simulink model "MultirotorModel"  (R2024b)
settings: Solver=VariableStepAuto  StartTime=0.0  StopTime=simTime  FixedStep=0.001  RelTol=1e-3  EnableMultiTasking=on
undefined symbols (not defined in the file): baseMission, bird_cycle, bird_end, bird_start, Controller, ctrl_mass, ctrl_thrust_perturbation_param, DiscIntNeverNeededParam, Dz, Earth, Gravity, initialConditions, Iz, mass_param, Nz, Pz, startFlightTime, UAVSampleTime, Vehicle, WGS84
libraries: slpidlib x10, uavalgslib x6, simulink x3, sharedutil x2, aerolibconvert2 x2, aerolibtransform2 x2, robotcorelib x1, uavutilslib x1, shared6dof x1, aerolibasang x1, sensorinslib x1
(part 3 of 3)

== system MultirotorModel/Inner Loop and Plant Model/High-FidelityModel/Control System/Controller/gravity feedforward//equilibrium thrust ==
  note: Derived from the work by Sertac Karaman and Fabian Riether
  note: ALTITUDE
  states_estim : Inport
  PosZ : Inport  Port=2
  Bus Selector1 : BusSelector  OutputSignals=pos_vel.z,pos_vel.vz
  D_z1 : Gain  Gain=3.5  ParamDataTypeStr=single  OutDataTypeStr=single  SaturateOnIntegerOverflow=on
  Discrete-Time Integrator : DiscreteIntegrator  SampleTime=UAVSampleTime  LimitOutput=on  UpperSaturationLimit=2  LowerSaturationLimit=-2  ICPrevOutput=DiscIntNeverNeededParam  ICPrevScaledInput=DiscIntNeverNeededParam
  I_pr : Gain  Gain=0.1
  MPC_THR_HOVER : Constant  Value=-Gravity*ctrl_mass  OutDataTypeStr=single
  P_z1 : Gain  Gain=0.4  ParamDataTypeStr=single  OutDataTypeStr=single  SaturateOnIntegerOverflow=on
  SaturationThrust1 : Saturate  UpperLimit=63  LowerLimit=-63  OutDataTypeStr=single
  SaturationThrust2 : Saturate  Commented=on  UpperLimit=4*Controller.totalThrustMaxRelative*Controller.motorsThrustPerMotorMax  LowerLimit=-4*Controller.totalThrustMaxRelative*Controller.motorsThrustPerMotorMax  OutDataTypeStr=single
  Scope : Scope
  Sum1 : Sum  Inputs=++-  OutDataTypeStr=single  AccumDataTypeStr=single  SaturateOnIntegerOverflow=on
  Sum2 : Sum  Inputs=+-|  OutDataTypeStr=single  AccumDataTypeStr=single  SaturateOnIntegerOverflow=on
  Sum5 : Sum  Inputs=++|  OutDataTypeStr=single  AccumDataTypeStr=single  SaturateOnIntegerOverflow=on
  altitude_cmd : Outport  VectorParamsAs1DForOutWhenUnconnected=off
  wires:
  I_pr/1 -> Discrete-Time Integrator/1
  Discrete-Time Integrator/1 -> Sum1/1
  D_z1/1 -> Sum1/3  "dz"
  Sum2/1 -> I_pr/1, P_z1/1  "pitch/roll error"
  Bus Selector1/2 -> D_z1/1  "<vz>"
  P_z1/1 -> Sum1/2
  states_estim/1 -> Bus Selector1/1
  Bus Selector1/1 -> Sum2/2  "<z>"
  PosZ/1 -> Sum2/1
  Sum1/1 -> Sum5/2
  Sum5/1 -> Scope/1, SaturationThrust1/1
  MPC_THR_HOVER/1 -> Sum5/1
  SaturationThrust1/1 -> altitude_cmd/1

== system MultirotorModel/Inner Loop and Plant Model/High-FidelityModel/Control System/Controller/thrustsToMotorCommands ==
  thrusts_refin : Inport
  MotorDirections : Gain  Gain=[1 -1 1 -1]
  Saturation5 : Saturate  Commented=on  UpperLimit=Vehicle.Motor.maxLimit  LowerLimit=Vehicle.Motor.minLimit
  ThrustToMotorCommand : Gain  Gain=-Vehicle.Motor.thrustToMotorCommand
  motors_cmdout : Outport  VectorParamsAs1DForOutWhenUnconnected=off
  wires:
  MotorDirections/1 -> motors_cmdout/1
  thrusts_refin/1 -> ThrustToMotorCommand/1
  ThrustToMotorCommand/1 -> MotorDirections/1

== system MultirotorModel/Inner Loop and Plant Model/High-FidelityModel/Plant Model/AC model/Applied Force Calculation ==
  gravity force : Inport  Unit=N
  Aerodynamic Forces : Inport  Port=2  Unit=N
  Motor Forces : Inport  Port=3  Unit=N
  Add1 : Sum  Inputs=+++
  Signal Specification : SignalSpecification  Dimensions=3
  External Forces : Outport  Unit=N  VectorParamsAs1DForOutWhenUnconnected=off
  wires:
  Add1/1 -> Signal Specification/1
  Motor Forces/1 -> Add1/3  "Motor Thrust"
  Aerodynamic Forces/1 -> Add1/2
  gravity force/1 -> Add1/1
  Signal Specification/1 -> External Forces/1

== system MultirotorModel/Inner Loop and Plant Model/High-FidelityModel/Plant Model/AC model/Drag Calculation ==
  Density : Inport  Unit=kg/m^3
  Vb : Inport  Port=2  Unit=m/second
  Drag Calc : Subsystem
  Gain3 : Gain  Gain=-1
  Product : Product  RndMeth=Zero
  Sign : Signum  ZeroCross=off
  Drag : Outport  Unit=N  VectorParamsAs1DForOutWhenUnconnected=off
  wires:
  Density/1 -> Drag Calc/1(Density)
  Sign/1 -> Gain3/1
  Drag Calc/1(drag) -> Product/1
  Gain3/1 -> Product/2
  Product/1 -> Drag/1  "xDrag"
  Vb/1 -> Sign/1, Drag Calc/2(vel)

== system MultirotorModel/Inner Loop and Plant Model/High-FidelityModel/Plant Model/AC model/Gravity Force Calculation ==
  DCMbe : Inport
  gravity : Inport  Port=2  Unit=m/s^2
  Gain1 : Gain  Gain=ctrl_mass
  Product : Product  Multiplication=Matrix(*)
  gravity force : Outport  Unit=N  VectorParamsAs1DForOutWhenUnconnected=off
  wires:
  gravity/1 -> Gain1/1
  Gain1/1 -> Product/2  "gravity force NED"
  Product/1 -> gravity force/1
  DCMbe/1 -> Product/1

== system MultirotorModel/Inner Loop and Plant Model/High-FidelityModel/Plant Model/AC model/Motor Forces and Torques ==
  Vb : Inport
  Density : Inport  Port=2
  pqr : Inport  Port=3
  Motor Commands : Inport  Port=4
  D1 : Constant  Value=[Vehicle.Airframe.xy -Vehicle.Airframe.xy Vehicle.Airframe.h]
  D2 : Constant  Value=[Vehicle.Airframe.xy Vehicle.Airframe.xy Vehicle.Airframe.h]
  D3 : Constant  Value=[-Vehicle.Airframe.xy Vehicle.Airframe.xy Vehicle.Airframe.h]
  D4 : Constant  Value=[-Vehicle.Airframe.xy -Vehicle.Airframe.xy Vehicle.Airframe.h]
  For Each Subsystem : Subsystem  TreatAsAtomicUnit=on
  MotorsToW : Subsystem
  Sum of Elements : Sum  Inputs=+  CollapseMode=Specified dimension  CollapseDim=2
  Sum of Elements1 : Sum  Inputs=+  CollapseMode=Specified dimension  CollapseDim=2
  Vector Concatenate : Concatenate  NumInputs=4  Mode=Multidimensional array  ConcatenateDimension=2
  Motor Forces : Outport  Unit=N  VectorParamsAs1DForOutWhenUnconnected=off
  Motor Torques : Outport  Port=2  Unit=N*m  VectorParamsAs1DForOutWhenUnconnected=off
  wires:
  D4/1 -> Vector Concatenate/4
  MotorsToW/1(omegas_datout) -> For Each Subsystem/4(w)
  Vector Concatenate/1 -> For Each Subsystem/5(D)
  For Each Subsystem/2(Moments) -> Sum of Elements1/1
  pqr/1 -> For Each Subsystem/3(Omega)
  Vb/1 -> For Each Subsystem/1(Vb)
  Motor Commands/1 -> MotorsToW/1(motors_datin)
  D1/1 -> Vector Concatenate/1
  D3/1 -> Vector Concatenate/3
  D2/1 -> Vector Concatenate/2
  Sum of Elements1/1 -> Motor Torques/1
  Density/1 -> For Each Subsystem/2(rho)
  Sum of Elements/1 -> Motor Forces/1
  For Each Subsystem/1(Forces) -> Sum of Elements/1

== system MultirotorModel/Inner Loop and Plant Model/High-FidelityModel/Plant Model/Bus setup/Generate GPS Data ==
  XYZ (NEU) : Inport
  "Vx, Vy, Vz" : Inport  Port=2
  DCM : Inport  Port=3
  GPS Model : sensorinslib/INS  MountingLocation=[0 0 0]  RollAccuracy=0.2  PitchAccuracy=0.2  YawAccuracy=1  PositionAccuracy=0.85  VelocityAccuracy=0.05  UseAccelAndAngVel=off  AccelerationAccuracy=0  AngularVelocityAccuracy=0  TimeInput=off  PositionErrorFactor=[0 0 0]  SeedDouble=67  SimulateUsing=Code generation
  Reshape : Reshape  OutputDimensionality=Customize  OutputDimensions=[1 3]
  Reshape1 : Reshape  OutputDimensionality=Customize  OutputDimensions=[1 3]
  "Scale and Assemble GPS Data " : Subsystem
  Terminator1 : Terminator
  Variant Source : VariantSource  VariantControlMode=label  LabelModeActiveChoice=Model
  Variant Source1 : VariantSource  VariantControlMode=label  LabelModeActiveChoice=Model
  GPSData : Outport  VectorParamsAs1DForOutWhenUnconnected=off
  wires:
  DCM/1 -> GPS Model/3
  "Vx, Vy, Vz"/1 -> Variant Source1/1, Reshape1/1
  XYZ (NEU)/1 -> Variant Source/1, Reshape/1
  GPS Model/3 -> Terminator1/1
  Reshape/1 -> GPS Model/1
  Reshape1/1 -> GPS Model/2
  "Scale and Assemble GPS Data "/1(Out1) -> GPSData/1
  GPS Model/1 -> Variant Source/2
  Variant Source1/1 -> "Scale and Assemble GPS Data "/2(Ve)
  GPS Model/2 -> Variant Source1/2
  Variant Source/1 -> "Scale and Assemble GPS Data "/1(Xe)

== system MultirotorModel/Guidance Logic/Full Guidance Logic/Guidance Stateflow/Guidance Mode Selector/GuidanceLogic.WP/Dist2WP/Subsystem ==
  V : Inport
  Dot Product1 : DotProduct  OutDataTypeStr=Inherit: Inherit via internal rule
  Product : Product  Inputs=*/
  Saturation : Saturate  UpperLimit=inf  LowerLimit=0.00001
  Sqrt : Sqrt
  V_unit : Outport
  wires:
  V/1 -> Dot Product1/2, Dot Product1/1, Product/1
  Sqrt/1 -> Product/2
  Dot Product1/1 -> Saturation/1
  Saturation/1 -> Sqrt/1
  Product/1 -> V_unit/1

== system MultirotorModel/Inner Loop and Plant Model/High-FidelityModel/Plant Model/AC model/Drag Calculation/Drag Calc ==
  Density : Inport  Unit=kg/m^3
  vel : Inport  Port=2  Unit=m/s
  Dynamic Pressure : aerolibasang/Dynamic Pressure
  Gain : Gain  Gain=[.25 .25]
  Mux1 : Mux  Inputs=2
  Product : Product  Inputs=3  RndMeth=Zero
  diameter : Constant  Value=0.65  SampleTime=0
  dragCoeff : Constant  Value=Vehicle.Airframe.Cdx  SampleTime=0
  drag : Outport  Unit=N  VectorParamsAs1DForOutWhenUnconnected=off
  wires:
  Product/1 -> drag/1
  dragCoeff/1 -> Product/3  "Cd"
  Dynamic Pressure/1 -> Product/1  "q"
  diameter/1 -> Gain/1, Mux1/2
  Mux1/1 -> Product/2  "S"
  Gain/1 -> Mux1/1
  vel/1 -> Dynamic Pressure/1
  Density/1 -> Dynamic Pressure/2

== system MultirotorModel/Inner Loop and Plant Model/High-FidelityModel/Plant Model/AC model/Motor Forces and Torques/For Each Subsystem ==
  Vb : Inport  PortDimensions=3
  rho : Inport  Port=2  PortDimensions=1
  Omega : Inport  Port=3
  w : Inport  Port=4  Partition=on  PartitionDimension=2  PartitionWidth=1  PartitionOffset=0
  D : Inport  Port=5  Partition=on  PartitionDimension=2  PartitionWidth=1  PartitionOffset=0
  For Each : ForEach  DisableCoverage=on
  RotorDynamics : Subsystem  TreatAsAtomicUnit=on
      mask init:
      | aeroicon('aeroblk');
      settings: RTWFcnNameOpts=Use subsystem name  RTWFileNameOpts=Use function name
  Forces : Outport  ConcatenationDimension=2  VectorParamsAs1DForOutWhenUnconnected=off
  Moments : Outport  Port=2  ConcatenationDimension=2  VectorParamsAs1DForOutWhenUnconnected=off
  wires:
  RotorDynamics/1(Fxyz) -> Forces/1
  RotorDynamics/2(Mxyz) -> Moments/1
  Vb/1 -> RotorDynamics/1(Vb)
  Omega/1 -> RotorDynamics/2(pqr)
  rho/1 -> RotorDynamics/3(rho)
  D/1 -> RotorDynamics/5(Arm)
  w/1 -> RotorDynamics/4(w)

== system MultirotorModel/Inner Loop and Plant Model/High-FidelityModel/Plant Model/AC model/Motor Forces and Torques/MotorsToW ==
  motors_datin : Inport
  Motordirections : Gain  Gain=[1 -1 1 -1]  ParamDataTypeStr=single  OutDataTypeStr=Inherit: Inherit via back propagation  SaturateOnIntegerOverflow=on
  Motordirections1 : Gain  Gain=[1 -1 1 -1]  ParamDataTypeStr=single  OutDataTypeStr=Inherit: Inherit via back propagation  SaturateOnIntegerOverflow=on
  Saturation1 : Saturate  UpperLimit=99999999999  LowerLimit=1  OutDataTypeStr=Inherit: Inherit via back propagation
  Saturation5 : Saturate  Commented=on  UpperLimit=Vehicle.Motor.maxLimit  LowerLimit=Vehicle.Motor.minLimit  OutDataTypeStr=Inherit: Inherit via back propagation
  Signed Sqrt : Sqrt  Operator=signedSqrt  OutDataTypeStr=Inherit: Inherit via back propagation
  motorsToW2_Gain : Gain  Gain=Vehicle.Motor.commandToW2Gain  ParamDataTypeStr=single  OutDataTypeStr=Inherit: Inherit via back propagation  SaturateOnIntegerOverflow=on
  omegas_datout : Outport  VectorParamsAs1DForOutWhenUnconnected=off
  wires:
  motorsToW2_Gain/1 -> Signed Sqrt/1
  Motordirections1/1 -> motorsToW2_Gain/1
  Signed Sqrt/1 -> omegas_datout/1
  motors_datin/1 -> Motordirections/1
  Motordirections/1 -> Saturation1/1
  Saturation1/1 -> Motordirections1/1

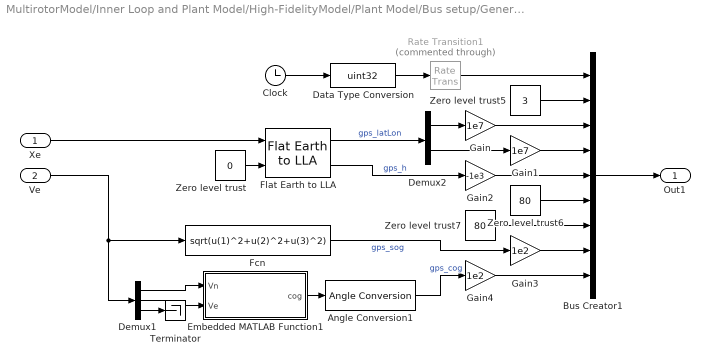
== system MultirotorModel/Inner Loop and Plant Model/High-FidelityModel/Plant Model/Bus setup/Generate GPS Data/Scale and Assemble GPS Data  ==
  Xe : Inport
  Ve : Inport  Port=2
  Angle Conversion1 : aerolibconvert2/Angle Conversion  IU=rad  OU=deg
  Bus Creator1 : BusCreator  Inputs=9  OutDataTypeStr=Bus: gps_raw_int  NonVirtualBus=on
      settings: InheritFromInputs=off
  Clock : Clock
      settings: AttributesFormatString=Decimation: %<Decimation>
  Data Type Conversion : DataTypeConversion  OutDataTypeStr=uint32  SaturateOnIntegerOverflow=off  RndMeth=Floor
  Demux1 : Demux  Outputs=3
  Demux2 : Demux  Outputs=2
  Embedded MATLAB Function1 : MATLAB Function  TreatAsAtomicUnit=on
  Fcn : Fcn  Expr=sqrt(u(1)^2+u(2)^2+u(3)^2)
  Flat Earth to LLA : aerolibtransform2/Flat Earth to LLA  units=Metric (MKS)  ptype=Earth (WGS84)  F=1/298.257223563  R=6378137  refPosPort=off  LL0=uavIC_latLon  psi=0
  Gain : Gain  Gain=1e7  OutDataTypeStr=int32
  Gain1 : Gain  Gain=1e7  OutDataTypeStr=int32
  Gain2 : Gain  Gain=-1e3  OutDataTypeStr=int32
  Gain3 : Gain  Gain=1e2  OutDataTypeStr=uint16
  Gain4 : Gain  Gain=1e2  OutDataTypeStr=uint16
  Rate Transition1 : RateTransition  Commented=through  OutPortSampleTime=0.005
  Terminator : Terminator
  Zero level trust : Constant  Value=0
      settings: AttributesFormatString=%<Value>
  Zero level trust5 : Constant  Value=3  OutDataTypeStr=uint8
      settings: AttributesFormatString=%<Value>
  Zero level trust6 : Constant  Value=80  OutDataTypeStr=uint16
      settings: AttributesFormatString=%<Value>
  Zero level trust7 : Constant  Value=80  OutDataTypeStr=uint16
      settings: AttributesFormatString=%<Value>
  Out1 : Outport
  wires:
  Demux2/1 -> Gain/1
  Gain/1 -> Bus Creator1/3
  Gain4/1 -> Bus Creator1/9
  Demux2/2 -> Gain1/1
  Embedded MATLAB Function1/1(cog) -> Angle Conversion1/1
  Rate Transition1/1 -> Bus Creator1/1
  Zero level trust6/1 -> Bus Creator1/6
  Gain3/1 -> Bus Creator1/8
  Clock/1 -> Data Type Conversion/1
  Ve/1 -> Demux1/1, Fcn/1
  Zero level trust7/1 -> Bus Creator1/7
  Data Type Conversion/1 -> Rate Transition1/1
  Demux1/2 -> Embedded MATLAB Function1/2(Ve)
  Zero level trust5/1 -> Bus Creator1/2
  Demux1/1 -> Embedded MATLAB Function1/1(Vn)
  Flat Earth to LLA/1 -> Demux2/1  "gps_latLon"
  Gain2/1 -> Bus Creator1/5
  Fcn/1 -> Gain3/1  "gps_sog"
  Gain1/1 -> Bus Creator1/4
  Flat Earth to LLA/2 -> Gain2/1  "gps_h"
  Zero level trust/1 -> Flat Earth to LLA/2
  Angle Conversion1/1 -> Gain4/1  "gps_cog"
  Demux1/3 -> Terminator/1
  Xe/1 -> Flat Earth to LLA/1
  Bus Creator1/1 -> Out1/1

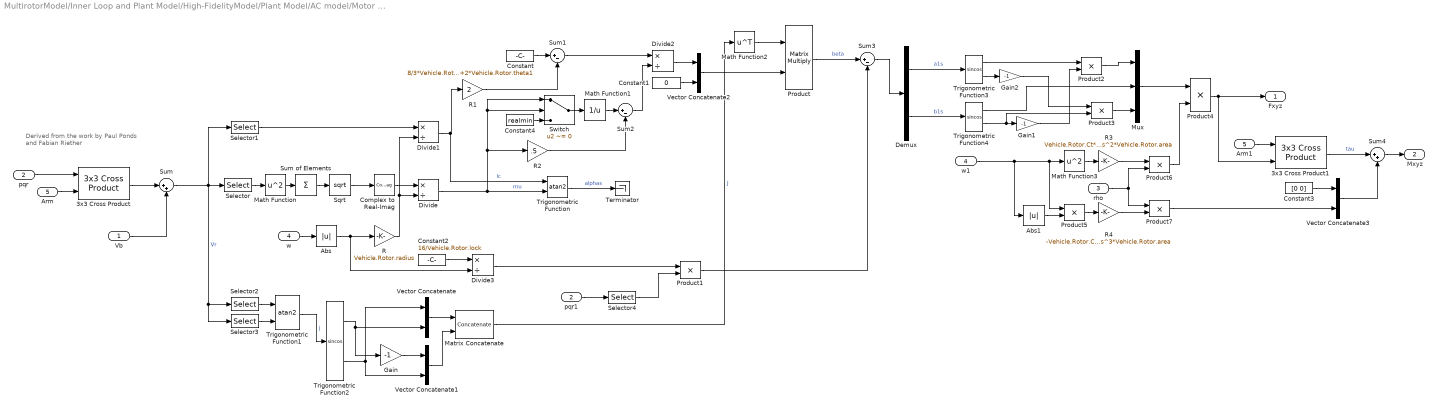
== system MultirotorModel/Inner Loop and Plant Model/High-FidelityModel/Plant Model/AC model/Motor Forces and Torques/For Each Subsystem/RotorDynamics ==
  note: Derived from the work by Paul Ponds
      | and Fabian Riether
  Vb : Inport  PortDimensions=3
  pqr : Inport  Port=2  PortDimensions=3
  rho : Inport  Port=3  PortDimensions=1
  w : Inport  Port=4  PortDimensions=[1 1]
  Arm : Inport  Port=5  PortDimensions=[3 1]
  3x3 Cross Product : sharedutil/3x3 Cross Product  aMode=aMode
  3x3 Cross Product1 : sharedutil/3x3 Cross Product  aMode=aMode
  Abs : Abs  SaturateOnIntegerOverflow=off
  Abs1 : Abs  SaturateOnIntegerOverflow=off
  Arm1 : InportShadow  Port=5  PortDimensions=[3 1]
  Complex to Real-Imag : ComplexToRealImag  Output=Real
  Constant : Constant  Value=8/3*Vehicle.Rotor.theta0+2*Vehicle.Rotor.theta1
  Constant1 : Constant  Value=0
  Constant2 : Constant  Value=16/Vehicle.Rotor.lock
  Constant3 : Constant  Value=[0 0]
  Constant4 : Constant  Value=realmin
  Demux : Demux  Outputs=2
  Divide{,1..3} (4 alike) : Product  Inputs=*/
  Gain : Gain  Gain=-1
  Gain1 : Gain  Gain=-1
  Gain2 : Gain  Gain=-1
  Math Function : Math  Operator=square  SignedPower=on
  Math Function1 : Math  Operator=reciprocal  SignedPower=on
  Math Function2 : Math  Operator=transpose  SignedPower=on
  Math Function3 : Math  Operator=square  SignedPower=on
  Matrix Concatenate : Concatenate  Mode=Multidimensional array  ConcatenateDimension=2
  Mux : Mux  Inputs=3
  Product : Product  Multiplication=Matrix(*)
  Product{1..7} (7 alike) : Product
  R : Gain  Gain=Vehicle.Rotor.radius
  R1 : Gain  Gain=2
  R2 : Gain  Gain=.5
  R3 : Gain  Gain=Vehicle.Rotor.Ct*Vehicle.Rotor.radius^2*Vehicle.Rotor.area
  R4 : Gain  Gain=-Vehicle.Rotor.Cq*Vehicle.Rotor.radius^3*Vehicle.Rotor.area
  Selector : Selector  InputPortWidth=3  IndexOptions=Index vector (dialog)  Indices=[1 2]  OutputSizes=1
  Selector1 : Selector  InputPortWidth=3  IndexOptions=Index vector (dialog)  Indices=[3]  OutputSizes=1
  Selector2 : Selector  InputPortWidth=3  IndexOptions=Index vector (dialog)  Indices=[2]  OutputSizes=1
  Selector3 : Selector  InputPortWidth=3  IndexOptions=Index vector (dialog)  Indices=[1]  OutputSizes=1
  Selector4 : Selector  InputPortWidth=3  IndexOptions=Index vector (dialog)  Indices=[2 1]  OutputSizes=1
  Sqrt : Sqrt  OutputSignalType=complex
  Sum : Sum  Inputs=|++
  Sum of Elements : Sum  Inputs=+
  Sum1 : Sum  Inputs=|+-
  Sum2 : Sum  Inputs=|+-
  Sum3 : Sum  Inputs=|+-
  Sum4 : Sum  Inputs=|++
  Switch : Switch  Criteria=u2 ~= 0  SaturateOnIntegerOverflow=off  InputSameDT=off
  Terminator : Terminator
  Trigonometric Function : Trigonometry  Operator=atan2
  Trigonometric Function1 : Trigonometry  Operator=atan2
  Trigonometric Function2 : Trigonometry  Operator=sincos
  Trigonometric Function3 : Trigonometry  Operator=sincos
  Trigonometric Function4 : Trigonometry  Operator=sincos
  Vector Concatenate{,1..3} (4 alike) : Concatenate
  pqr1 : InportShadow  Port=2  PortDimensions=3
  w1 : InportShadow  Port=4  PortDimensions=[1 1]
  Fxyz : Outport  PortDimensions=[3 1]  VectorParamsAs1DForOutWhenUnconnected=off
  Mxyz : Outport  Port=2  PortDimensions=[3 1]  VectorParamsAs1DForOutWhenUnconnected=off
  wires:
  Complex to Real-Imag/1 -> Divide/1
  Sqrt/1 -> Complex to Real-Imag/1
  Constant4/1 -> Switch/3
  Switch/1 -> Math Function1/1
  Product1/1 -> Sum3/2
  rho/1 -> Product7/1, Product6/2
  Product7/1 -> Vector Concatenate3/2
  Product6/1 -> Product4/2
  Sum4/1 -> Mxyz/1
  3x3 Cross Product1/1 -> Sum4/1  "tau"
  Product4/1 -> Fxyz/1, 3x3 Cross Product1/2
  Arm1/1 -> 3x3 Cross Product1/1
  Vector Concatenate3/1 -> Sum4/2
  Constant3/1 -> Vector Concatenate3/1
  R4/1 -> Product7/2
  Product5/1 -> R4/1
  Abs1/1 -> Product5/2
  R3/1 -> Product6/1
  Mux/1 -> Product4/1
  Gain2/1 -> Product3/1
  Product3/1 -> Mux/3
  Trigonometric Function3/2 -> Gain2/1
  Trigonometric Function4/1 -> Mux/2
  Product2/1 -> Mux/1
  Trigonometric Function3/1 -> Product2/1
  Gain1/1 -> Product2/2
  Trigonometric Function4/2 -> Gain1/1, Product3/2
  Demux/2 -> Trigonometric Function4/1  "b1s"
  Demux/1 -> Trigonometric Function3/1  "a1s"
  Sum3/1 -> Demux/1
  Math Function3/1 -> R3/1
  w1/1 -> Math Function3/1, Product5/1, Abs1/1
  Divide3/1 -> Product1/1
  Abs/1 -> R/1, Divide3/2
  Selector4/1 -> Product1/2
  pqr1/1 -> Selector4/1
  Constant2/1 -> Divide3/1
  Product/1 -> Sum3/1  "beta"
  Math Function2/1 -> Product/1
  Vector Concatenate2/1 -> Product/2
  Constant1/1 -> Vector Concatenate2/2
  Divide2/1 -> Vector Concatenate2/1
  Sum2/1 -> Divide2/2
  R2/1 -> Sum2/2
  Math Function1/1 -> Sum2/1
  Sum1/1 -> Divide2/1
  R1/1 -> Sum1/2
  Constant/1 -> Sum1/1
  Matrix Concatenate/1 -> Math Function2/1  "J"
  Vector Concatenate1/1 -> Matrix Concatenate/2
  Vector Concatenate/1 -> Matrix Concatenate/1
  Trigonometric Function2/1 -> Gain/1, Vector Concatenate/2
  Gain/1 -> Vector Concatenate1/1
  Trigonometric Function2/2 -> Vector Concatenate/1, Vector Concatenate1/2
  Trigonometric Function1/1 -> Trigonometric Function2/1  "j"
  Selector3/1 -> Trigonometric Function1/2
  Selector2/1 -> Trigonometric Function1/1
  Trigonometric Function/1 -> Terminator/1  "alphas"
  Divide1/1 -> Trigonometric Function/1, R1/1  "lc"
  Selector1/1 -> Divide1/1
  Divide/1 -> Trigonometric Function/2, Switch/1, Switch/2, R2/1  "mu"
  R/1 -> Divide/2, Divide1/2
  w/1 -> Abs/1
  Arm/1 -> 3x3 Cross Product/2
  pqr/1 -> 3x3 Cross Product/1
  Sum of Elements/1 -> Sqrt/1
  Math Function/1 -> Sum of Elements/1
  Selector/1 -> Math Function/1
  Sum/1 -> Selector/1, Selector1/1, Selector2/1, Selector3/1  "Vr"
  Vb/1 -> Sum/2
  3x3 Cross Product/1 -> Sum/1

== matlab function MultirotorModel/Guidance Logic/Full Guidance Logic/Guidance Stateflow/Guidance Mode Selector/GuidanceLogic.Land.ToLand/MATLAB Function ==
  data: FromWP input Bus: uavPathManagerBus size=1; wps output; ToWP input Bus: uavPathManagerBus size=1
function wps = getLandingWaypoint(FromWP, ToWP)

persistent outWPS

if isempty(outWPS)
    outWPS = single(zeros(2,4));
end

outWPS(1,:) = [FromWP.position' FromWP.params(4)];
outWPS(2,:) = [ToWP.position(1:2)' -15 ToWP.params(4)];

wps = outWPS;

== matlab function MultirotorModel/Guidance Logic/Full Guidance Logic/Guidance Stateflow/Guidance Mode Selector/GuidanceLogic.WP/MATLAB Function ==
  data: FromWP input Bus: uavPathManagerBus size=1; wps output; ToWP input Bus: uavPathManagerBus size=1
function wps = getWaypointMission(FromWP, ToWP)

persistent outWPS

if isempty(outWPS)
    outWPS = single(zeros(2,4));
end

outWPS(1,:) = [FromWP.position' FromWP.params(4)];
outWPS(2,:) = [ToWP.position' ToWP.params(4)];

% for ii=1:2
%     outWPS(ii,1:3) = GCSMission(ii).position';
%     outWPS(ii,4) = GCSMission(ii).params(4);
% end

wps = outWPS;

== matlab function MultirotorModel/Guidance Logic/Obstacle Avoidance3D/MATLAB Function ==
  data: mission input; Steer input size=[5 1]; y output; UAVState input; DTD output; needHover output
function [y, DTD, needHover] = computeLPWaypoints(mission, Steer,UAVState)
%#codegen

Wp1 = [mission(1).position' mission(1).params(4)];
Wp2x = mission(2).position(1);
Wp2y = mission(2).position(2);
needHover = false;

% Follow obstacle avoidance steer direction when UAV is above 5 meters
% above ground
if (~any(isnan(Steer)) && (UAVState.z < -5))
    if (Steer(5) == 0)
        % Compute look ahead point 6 meters along the steering direction
        LAP_local = 6*Steer(2:4)';
        % Follow yaw command from obstacle avoidance
        yaw = Steer(1);
        LAP = [LAP_local yaw] + [UAVState.x, UAVState.y, UAVState.z, 0];
        if(isnan(LAP(4)))
            LAP(4) = 0;
        end

        y = [ Wp1(1,:) ; LAP ; Wp2x , Wp2y , 0 , LAP(4) ];
        DTD = norm([Wp2x Wp2y] - LAP(1:2));
    else
        % Rotate in place
        y = [ Wp1(1,:) ; UAVState.x, UAVState.y, UAVState.z Steer(1); Wp2x , Wp2y , 0 , Steer(1) ];
        DTD = norm([Wp2x Wp2y] - [UAVState.x, UAVState.y]);
        needHover = true;
    end
    
else
    % If there is no good steer direction or UAV is too low, fly up
    y = [ Wp1(1,:) ; UAVState.x , UAVState.y , UAVState.z-2 , 0 ; Wp2x , Wp2y , 0 , 0 ];
    DTD = norm([Wp2x Wp2y] - [UAVState.x, UAVState.y]);
end

if(DTD<5)
    % When close to target point, switch to landing
    y = [ Wp1(1,:) ; Wp2x , Wp2y, -11 , 0 ; Wp2x , Wp2y , -1 , 0 ];
end


end

== matlab function MultirotorModel/Guidance Logic/Full Guidance Logic/Guidance Stateflow/Guidance Mode Selector/GuidanceLogic.WP/APF_Avoidance ==
  data: pose input; correctedCourse output; desiredCourse input; desiredYaw input; obstacle input; correctedYaw output
function [correctedCourse, correctedYaw] = APF_Avoidance(pose, desiredCourse, desiredYaw, obstacle)
% APF_Avoidance: Artificial Potential Field avoidance controller
%
% Inputs:
%   pose: [x, y, z] position (single or double)
%   desiredCourse: angle (rad)
%   desiredYaw: angle (rad)
%   obstacle: [1 x 3] vector, obstacle position
%
% Outputs:
%   correctedCourse: adjusted course angle (rad)
%   correctedYaw: adjusted yaw angle (rad)

% Ensure consistent type
typeRef = pose(1);

% Parameters (tune as needed)
k_att = cast(1, 'like', typeRef);       % attractive gain
k_rep = cast(2, 'like', typeRef);       % repulsive gain
rep_range = cast(5, 'like', typeRef);   % influence range (meters)
min_dist = cast(0.1, 'like', typeRef);  % avoid div by zero

% Compute attractive force
att_x = k_att * cos(desiredCourse);
att_y = k_att * sin(desiredCourse);

% Initialize repulsive force
rep_x = zeros(1, 'like', typeRef);
rep_y = zeros(1, 'like', typeRef);

% Process single obstacle
pos2D = pose(1:2);
obs2D = obstacle(1:2);
vec = pos2D - obs2D;
dist = sqrt(vec(1)^2 + vec(2)^2);

if dist < rep_range && dist > min_dist
    repulse = k_rep * (1/dist - 1/rep_range) / (dist^2);
    rep_x = repulse * (vec(1)/dist);
    rep_y = repulse * (vec(2)/dist);
end

% Combine forces
sum_x = att_x + rep_x;
sum_y = att_y + rep_y;

% Compute corrected course
correctedCourse = atan2(sum_y, sum_x);
correctedYaw = correctedCourse; % match yaw to course, can be split if needed

end

== matlab function MultirotorModel/Guidance Logic/Full Guidance Logic/Guidance Stateflow/Guidance Mode Selector/GuidanceLogic.Land.ToLand/APF_Avoidance ==
  data: pose input; correctedCourse output; desiredCourse input; obstacle input; correctedYaw output; dbg_dist output; dbg_inRange output; dbg_repulse output; vel_self input; vel_obs input
function [correctedCourse, correctedYaw, dbg_dist, dbg_inRange, dbg_repulse] = APF_Avoidance(pose, desiredCourse, obstacle, vel_self, vel_obs)
% APF_Avoidance: Artificial Potential Field avoidance controller with dynamic obstacle handling
%
% Inputs:
%   pose:        [x, y, z] position of drone
%   desiredCourse: desired heading (rad)
%   obstacle:    [x, y, z] position of obstacle
%   vel_self:    [vx, vy] velocity of the drone
%   vel_obs:     [vx, vy] velocity of the obstacle
%
% Outputs:
%   correctedCourse: adjusted course angle (rad)
%   correctedYaw:    matched yaw (rad)
%   dbg_*:           debug outputs for analysis

% Ensure type safety
typeRef = pose(1);
dbg_repulse = cast(0, 'like', typeRef);

persistent avoid_dir prevCourse
if isempty(avoid_dir)
    avoid_dir = cast(NaN, 'like', typeRef);
end
if isempty(prevCourse)
    prevCourse = desiredCourse;
end

% Parameters
k_att = cast(1, 'like', typeRef);
k_rep = cast(50, 'like', typeRef);
rep_range = cast(20, 'like', typeRef);
min_dist = cast(0.1, 'like', typeRef);
early_buffer = cast(5, 'like', typeRef);
exit_range = rep_range + 10;

max_rate = deg2rad(25);  % 25 deg/sec limit
Ts = 0.05;               % timestep
max_delta = max_rate * Ts;

% Attractive force
att_x = k_att * cos(desiredCourse);
att_y = k_att * sin(desiredCourse);

% Distance and vector
vec = [pose(1) - obstacle(1), pose(2) - obstacle(2)];
dist = sqrt(sum(vec.^2));
dbg_dist = cast(dist, 'like', typeRef);
vec_xy_norm = vec / max(dist, min_dist);
travel_dir = [cos(desiredCourse), sin(desiredCourse)];
closing_in = dot(-vec_xy_norm, travel_dir) > 0;

% Reset avoidance decision if far
if dist > exit_range
    avoid_dir = cast(NaN, 'like', typeRef);  % only reset far away
end

% Influence check
inRange = dist < (rep_range + early_buffer) && dist > min_dist && closing_in;
dbg_inRange = cast(inRange, 'like', typeRef);

rep_x = cast(0, 'like', typeRef);
rep_y = cast(0, 'like', typeRef);

if inRange
    repulse = k_rep * (rep_range - dist) / rep_range;
    dbg_repulse = cast(repulse, 'like', typeRef);

    % Compute relative velocity
    rel_vel = vel_self(1:2) - vel_obs(1:2);
    rel_speed = norm(rel_vel);
    rel_dir = rel_vel / max(rel_speed, min_dist);

    % Adjust repulsion strength based on approach speed
    speed_factor = cast(1 + 2 * dot(vec_xy_norm, rel_dir), 'like', typeRef);
    repulse = repulse * max(speed_factor, 0.1); % prevent negative or 0

    vec_angle = atan2(vec_xy_norm(2), vec_xy_norm(1));
    angle_diff = atan2(sin(vec_angle - desiredCourse), cos(vec_angle - desiredCourse));
    
    if abs(angle_diff) < deg2rad(20) && isnan(avoid_dir)
        % Decide avoidance direction based on relative motion
        % If relative velocity is mostly horizontal, bias left/right based on y-component
        if abs(rel_vel(2)) > abs(rel_vel(1))
            avoid_dir = cast(sign(rel_vel(2)), 'like', typeRef);  % go opposite to vertical approach
        else
            % Use position-based bias if motion is nearly head-on
            obs_vec = obstacle(1:2) - pose(1:2);
            side_sign = sign(travel_dir(1)*obs_vec(2) - travel_dir(2)*obs_vec(1));
            avoid_dir = cast(side_sign, 'like', typeRef);
        end
    end

    % Avoid direction: lock if close
    if isnan(avoid_dir) || (dist < 8 && closing_in)
        obs_vec = obstacle(1:2) - pose(1:2);
        side_sign = sign(travel_dir(1)*obs_vec(2) - travel_dir(2)*obs_vec(1));
        avoid_dir = cast(side_sign, 'like', typeRef);
    end

    % Perpendicular direction for deflection
    perp = [-travel_dir(2), travel_dir(1)];
    rep_force = repulse * avoid_dir * perp;

    rep_x = rep_force(1);
    rep_y = rep_force(2);
end

% Combine forces
sum_x = att_x + rep_x;
sum_y = att_y + rep_y;

% Raw course
rawCourse = atan2(sum_y, sum_x);

% Rate-limited heading
delta = atan2(sin(rawCourse - prevCourse), cos(rawCourse - prevCourse));
delta = min(max(delta, -max_delta), max_delta);
correctedCourse = prevCourse + delta;
correctedCourse = mod(correctedCourse + pi, 2*pi) - pi;

% Update state
prevCourse = correctedCourse;
correctedYaw = correctedCourse;

end

== matlab function MultirotorModel/Animation/Bird Motion/BirdMotion ==
  data: t input; out output double size=[1 6]; start_pt input; end_pt input; cycle_time input
function out = BirdMotion(t, start_pt, end_pt, cycle_time)
% BirdMotion: bird flies back and forth between two points with wiggle
% Outputs: [x y z vx vy vz]

% Row vectors
start_pt = reshape(start_pt, 1, 3);
end_pt   = reshape(end_pt, 1, 3);

% Total direction vector and distance
delta = end_pt - start_pt;

% Phase: triangular wave [0–1–0–1...] over full cycle
half_cycle = cycle_time / 2;
phase = abs(mod(t, cycle_time) / half_cycle - 1);  % 0→1→0→...

% Position interpolation
pos_interp = start_pt + delta * phase;

% Wiggle for realism
amp  = [0.5, 0.5, 0.2];         % wiggle amplitude
freq = [1.0, 1.2, 0.8];         % wiggle frequency
wiggle = amp .* sin(freq * t); % element-wise

% Final position
pos = pos_interp + wiggle;

% Velocity: direction depends on phase direction
% If going 0→1, vel = +delta/half_cycle; if 1→0, vel = -delta/half_cycle
dir_sign = sign(cos(2 * pi * t / cycle_time));  % +1 or -1
vel = dir_sign * delta / half_cycle;

% Output
out = [pos, vel];
end

== matlab function MultirotorModel/Inner Loop and Plant Model/Low-FidelityModel/Assemble UAV State Bus/Generate GPS Data/Embedded MATLAB Function1 ==
  data: cog output; Vn input; Ve input
function cog = getCOG(Vn, Ve)
% This block supports an embeddable subset of the MATLAB language.
% See the help menu for details. 

cog = atan2(Ve,Vn);
if cog < 0;
    cog = cog + 2*pi;
end

== matlab function MultirotorModel/Guidance Logic/Obstacle Avoidance/MATLAB Function ==
  data: mission input; Steer input; y output; UAVState input
function y = computeLPWaypoints(mission, Steer,UAVState)
%#codegen

Wp1 = [mission(1).position' mission(1).params(4)];
Wp2x = mission(2).position(1);
Wp2y = mission(2).position(2);

if(~isnan(Steer))
    
    LAP_local = 6*[cos(Steer), sin(Steer)];
    LAP = [ LAP_local(1)+ UAVState.x , LAP_local(2) + UAVState.y , -11 , Steer];   
    if(isnan(LAP(4)))
        LAP(4) = 0;
    end
   
    y = [ Wp1(1,:) ; LAP ; Wp2x , Wp2y , 0 , Steer ];    
    DTD = sqrt( (LAP(1) - Wp2x)^2 + (LAP(2)-Wp2y)^2);  
    
else
    y = [ Wp1(1,:) ; UAVState.x , UAVState.y , UAVState.z-2 , 0 ; Wp2x , Wp2y , 0 , 0 ];
    DTD = sqrt( (UAVState.x - Wp2x)^2 + (UAVState.y-Wp2y)^2);
end

if(DTD<5)
    y = [ Wp1(1,:) ; Wp2x , Wp2y, -11 , 0 ; Wp2x , Wp2y , 0 , 0 ];
end


end

== matlab function MultirotorModel/Guidance Logic/Full Guidance Logic/Guidance Stateflow/Bird Motion/BirdMotion ==
  data: t input; out output double size=[1 6]; start_pt input; end_pt input; cycle_time input
function out = BirdMotion(t, start_pt, end_pt, cycle_time)
% BirdMotion: bird flies back and forth between two points with wiggle
% Outputs: [x y z vx vy vz]

% Row vectors
start_pt = reshape(start_pt, 1, 3);
end_pt   = reshape(end_pt, 1, 3);

% Total direction vector and distance
delta = end_pt - start_pt;

% Phase: triangular wave [0–1–0–1...] over full cycle
half_cycle = cycle_time / 2;
phase = abs(mod(t, cycle_time) / half_cycle - 1);  % 0→1→0→...

% Position interpolation
pos_interp = start_pt + delta * phase;

% Wiggle for realism
amp  = [0.5, 0.5, 0.2];         % wiggle amplitude
freq = [1.0, 1.2, 0.8];         % wiggle frequency
wiggle = amp .* sin(freq * t); % element-wise

% Final position
pos = pos_interp + wiggle;

% Velocity: direction depends on phase direction
% If going 0→1, vel = +delta/half_cycle; if 1→0, vel = -delta/half_cycle
dir_sign = sign(cos(2 * pi * t / cycle_time));  % +1 or -1
vel = dir_sign * delta / half_cycle;

% Output
out = [pos, vel];
end

== matlab function MultirotorModel/Inner Loop and Plant Model/Low-FidelityModel/Position and Acceleration Control/Attitude Control/Multirotor Acceleration Control ==
  data: acc input; roll output; pitch output; yaw input; Gravity parameter
function [roll, pitch] = accControl(acc, yaw, Gravity)

    xddot = acc(1);
    yddot = acc(2);
    zddot = acc(3);
    
    pitch = atan2((-xddot*cos(yaw)-yddot*sin(yaw)), ( -zddot + Gravity));
    roll = atan2(((-xddot*sin(yaw)+yddot*cos(yaw))*cos(pitch)), (-zddot+Gravity));
    
end

== matlab function MultirotorModel/Inner Loop and Plant Model/Low-FidelityModel/Position and Acceleration Control/Attitude Control/Multirotor Thrust Control ==
  data: acc input; pitch input; thrust output; roll input; mass_param parameter; Gravity parameter
function thrust  = thrustControl(acc, pitch, roll, mass_param, Gravity)

    zddot = acc(3);
    
    thrust = mass_param*(-zddot+Gravity)/(cos(pitch)*cos(roll));
end

== matlab function MultirotorModel/Inner Loop and Plant Model/High-FidelityModel/Control System/Controller/Position Controller/Position error transformation (Earth to Body frame) ==
  data: yaw input; xy_err_earth input; xy_err_body output
function xy_err_body = LTP2B2D(yaw,xy_err_earth)

transformation = [cos(yaw), sin(yaw); -sin(yaw),  cos(yaw)];
xy_err_body = transformation * xy_err_earth;


end

== matlab function MultirotorModel/Inner Loop and Plant Model/High-FidelityModel/Control System/Controller/Position Controller/Velocity error transformation (Earth to Body frame) ==
  data: yaw input; xy_err_earth input; xy_err_body output
function xy_err_body = LTP2B2D(yaw,xy_err_earth)

transformation = [cos(yaw), sin(yaw); -sin(yaw),  cos(yaw)];
xy_err_body = transformation * xy_err_earth;


end

== matlab function MultirotorModel/Inner Loop and Plant Model/High-FidelityModel/Control System/Controller/Yaw Controller/MATLAB Function ==
  data: u input; y output
function y = wrapYaw(u)
%u error in rad in -2pi to 2pi

if (u>pi)
    y = u-2*pi;
elseif(u<-pi)
    y = u +2*pi;
else
    y=u;
end

== matlab function MultirotorModel/Inner Loop and Plant Model/High-FidelityModel/Control System/Controller/Yaw Controller/MATLAB Function1 ==
  data: u input; y output
function y = wrapYaw(u)
%u error in rad in -2pi to 2pi

if (u>pi)
    y = u-2*pi;
elseif(u<-pi)
    y = u +2*pi;
else
    y=u;
end

== matlab function MultirotorModel/Inner Loop and Plant Model/High-FidelityModel/Plant Model/Bus setup/Generate GPS Data/Scale and Assemble GPS Data /Embedded MATLAB Function1 ==
  data: cog output; Vn input; Ve input
function cog = getCOG(Vn, Ve)
% This block supports an embeddable subset of the MATLAB language.
% See the help menu for details. 

cog = atan2(Ve,Vn);
if cog < 0;
    cog = cog + 2*pi;
end

== stateflow chart MultirotorModel/Guidance Logic/Full Guidance Logic/Guidance Stateflow/Guidance Mode Selector ==
  settings: updateMethod=DISCRETE  sampleTime=UAVSampleTime*4
  state GuidanceLogic
    state OnGround
    state Takeoff
    state WP
    state Orbit
    state Land
      state ToLand
      state Descend
      (default) -> ToLand
      ToLand -> Descend : [norm(Pose(1:2)-ToWP.position(1:2)) <= 5]
    (default) -> OnGround
    OnGround -> (junction 5) : [startFlight==1]
    Takeoff -> WP : [Pose(3) <= ToWP.position(3)]{Status = 1;}
    GuidanceLogic -> (junction 5) : [hasChanged(mode)]
    (junction 5) -> Takeoff [order 1] : [mode == 1]
    (junction 5) -> (junction 12) [order 2]
    (junction 12) -> WP [order 1] : [mode==2]
    (junction 12) -> (junction 17) [order 2]
    WP -> GuidanceLogic [commented out] : [Pose(2) < -110 || Pose(1) > -115 || ((Pose(1) < -125 && Pose(2) > -95))] {Status = 2;}
    (junction 17) -> Orbit [order 1] : [mode==3]
    (junction 17) -> (junction 22) [order 2]
    (junction 22) -> Land
    Land -> GuidanceLogic : [Pose(3)>=-1]{Status = 2;}
  (default) -> GuidanceLogic
  data: sf_internal_action_state_placeholder_data local double size=1 =0; sf_internal_action_state_placeholder_data local double size=1 =0; sf_internal_action_state_placeholder_data local double size=1 =0; sf_internal_action_state_placeholder_data local double size=1 =0; sf_internal_action_state_placeholder_data local double size=1 =0; mode input; ToWP input Bus: uavPathManagerBus; InnerLoopCmds output Bus: innerLoopCmdsBus; Status output uint8; FromWP input Bus: uavPathManagerBus; Pose input; startFlight input; GdncMode output Enum: GdncModeType; BirdPos input; DroneVel input; BirdVel input
